simulink model "ros_deneme"  (R2021a)
settings: Solver=ode113  StartTime=0.0  StopTime=10  FixedStep=0.1  MaxStep=0.1  RelTol=1e-3
model workspace (MAT data in the model file):
  SL_ROS_VariableLengthArrays_MaxSizes.CommonInfo.ArrayTruncateAction = 'EmitWarning'
  SL_ROS_VariableLengthArrays_MaxSizes.MsgTypeMap = containers.Map
  SL_ROS_VariableLengthArrays_MaxSizes.MsgTypeMap.serialization.keys = {'sensor_msgs/Image'}
  SL_ROS_VariableLengthArrays_MaxSizes.MsgTypeMap.serialization.values{1}(1).PropertyName = 'Data'
  SL_ROS_VariableLengthArrays_MaxSizes.MsgTypeMap.serialization.values{1}(1).DataType = 'uint8'
  SL_ROS_VariableLengthArrays_MaxSizes.MsgTypeMap.serialization.values{1}(1).MaxLength = 921600
  SL_ROS_VariableLengthArrays_MaxSizes.MsgTypeMap.serialization.values{1}(2).PropertyName = 'Encoding'
  SL_ROS_VariableLengthArrays_MaxSizes.MsgTypeMap.serialization.values{1}(2).DataType = 'uint8'
  SL_ROS_VariableLengthArrays_MaxSizes.MsgTypeMap.serialization.values{1}(2).MaxLength = 128
  SL_ROS_VariableLengthArrays_MaxSizes.MsgTypeMap.serialization.uniformity = 0
  SL_ROS_VariableLengthArrays_MaxSizes.MsgTypeMap.serialization.keyType = 'char'
  SL_ROS_VariableLengthArrays_MaxSizes.MsgTypeMap.serialization.valueType = 'any'
values from neighbouring files (symbols this model uses):
  A_Lat_F = [ Yb/V        Yp/V            (Yr/V)-1       9.81/V ... (first row only)    [modelCode.m]
  A_Long_F = [ Xu            Xw            0            -9.81 ... (first row only)    [modelCode.m]
  B_Lat_F = [ 0           Y_trim_r/V ... (first row only)    [modelCode.m]
  B_Long_F = [ Z_trim_e ... (first row only)    [modelCode.m]
  V = 85    [modelCode.m]
undefined symbols (not defined in the file or in its folder): ModelName, ModelName_SL_Info, Pose
libraries: robotlib x6, pid_lib x3, robotcorelib x1
settings Model: Creator=ommda  LastModifiedBy=lambdavary
settings SolverCC: AlgebraicLoopSolver=TrustRegion
settings DebuggingCC: SFMachineParentedDataDiag=warning

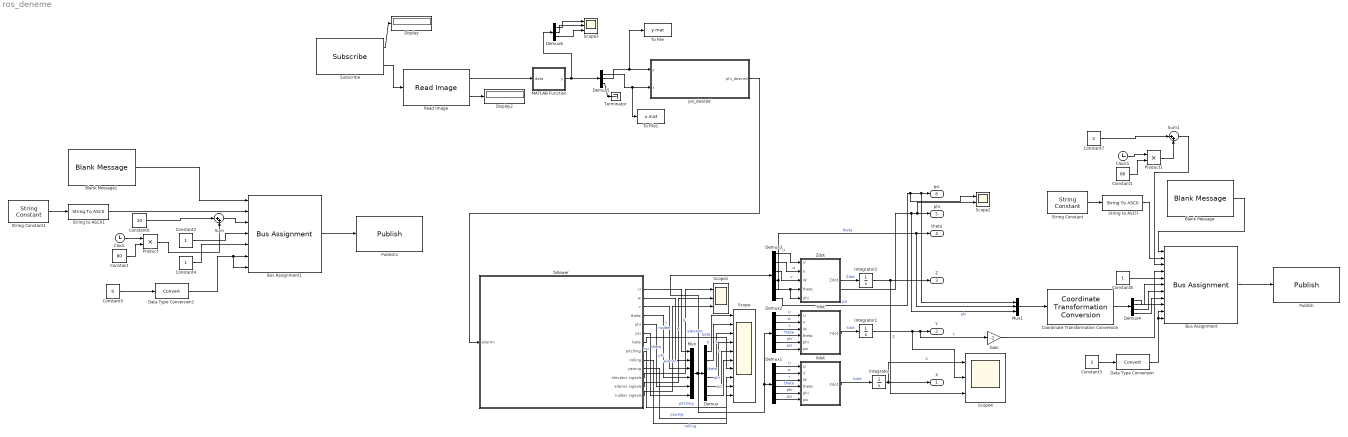
== system ros_deneme ==
  Blank Message : robotlib/Blank Message  messageClass=Message  entityType=gazebo_msgs/ModelState  messageType=gazebo_msgs/ModelState  SampleTime=inf  legacyBusStruct=off
  Blank Message1 : robotlib/Blank Message  messageClass=Message  entityType=gazebo_msgs/ModelState  messageType=gazebo_msgs/ModelState  SampleTime=inf  legacyBusStruct=off
  Bus Assignment : BusAssignment  AssignedSignals=ModelName,Pose.Position.X,Pose.Position.Y,Pose.Position.Z,Pose.Orientation.X,Pose.Orientation.Y,Pose.Orientation.Z,Pose.Orientation.W,ModelName_SL_Info.CurrentLength,ModelName_SL_Info.ReceivedLength
  Bus Assignment1 : BusAssignment  AssignedSignals=ModelName,Pose.Position.X,Pose.Position.Y,Pose.Position.Z,ModelName_SL_Info.CurrentLength,ModelName_SL_Info.ReceivedLength
  Clock : Clock
  Clock1 : Clock
  Constant : Constant  Value=80
  Constant1 : Constant  Value=80
  Constant2 : Constant
  Constant3 : Constant  Value=3
  Constant4 : Constant
  Constant5 : Constant  Value=6
  Constant6 : Constant  Value=10
  Constant7 : Constant  Value=2
  Constant8 : Constant
  Coordinate Transformation Conversion : robotcorelib/Coordinate Transformation Conversion  InputRepresentation=Euler Angles  InputEulerSequence=ZYX  ShowTrVecInputPort=on  OutputRepresentation=Quaternion  OutputEulerSequence=ZYX  ShowTrVecOutputPort=on  SimulateUsing=Interpreted execution
      settings: SourceProductBaseCode=NV,RO,RR,UV
  Data Type Conversion : DataTypeConversion
  Data Type Conversion1 : DataTypeConversion
  Demux{,1..3} (4 alike) : Demux  Outputs=6
  Demux4 : Demux
  Demux5 : Demux  Outputs=3
  Demux6 : Demux  Outputs=3
  Display : Display
  Display2 : Display
  Gain : Gain  Gain=-1
  Integrator : Integrator
  Integrator1 : Integrator
  Integrator2 : Integrator
  MATLAB Function : MATLAB Function  TreatAsAtomicUnit=on
  Mux : Mux  Inputs=6
  Mux1 : Mux  Inputs=3
  Product : Product
  Product1 : Product
  Publish : robotlib/Publish  topicSource=Select from ROS network  topic=/gazebo/set_model_state  messageType=gazebo_msgs/ModelState  legacyBusStruct=off  messageQueueLength=1
  Publish1 : robotlib/Publish  topicSource=Select from ROS network  topic=/gazebo/set_model_state  messageType=gazebo_msgs/ModelState  legacyBusStruct=off  messageQueueLength=1
  Read Image : robotlib/Read Image  MaximumImageSize=[480, 640]  ImageEncoding=rgb8  ShowAlphaOutput=off  ShowErrorCodeOutput=on  VariableSizeOutputs=off
      settings: SourceProductBaseCode=RR
  Scope : Scope  NumInputPorts=10
  Scope1 : Scope  NumInputPorts=3
  Scope2 : Scope  NumInputPorts=2
  Scope3 : Scope  NumInputPorts=3
  Scope4 : Scope  NumInputPorts=3
  String Constant : StringConstant  String="\"yau\""
  String Constant1 : StringConstant  String="\"tanker\""
  String to ASCII : StringToASCII  OutputVectorSize=128
  String to ASCII1 : StringToASCII  OutputVectorSize=128
  Subscribe : robotlib/Subscribe  topicSource=Select from ROS network  topic=/camera/image_raw  messageType=sensor_msgs/Image  SampleTime=-1  legacyBusStruct=off  messageQueueLength=1
  Sum : Sum  Inputs=|++
  Sum1 : Sum  Inputs=|++
  Terminator : Terminator
  To File : ToFile  Filename=y.mat
  To File1 : ToFile  Filename=x.mat
  Xdot : Subsystem
  Ydot : Subsystem
  Zdot : Subsystem
  follower : Subsystem
      mask Display: image('D:\Downloads\1200px-Yaw_Axis_Corrected.svg.png'); % Use "Edit Image" on toolstrip to change.
  psi_desired : Subsystem
  X : Outport
  Y : Outport  Port=2
  Z : Outport  Port=3
  theta : Outport  Port=4
  phi : Outport  Port=5
  psi : Outport  Port=6
  wires:
  Demux2/3 -> Ydot/3(W)  "v"
  Demux2/2 -> Ydot/2(V)  "w"
  follower/3(v) -> Mux/3  "v"
  Zdot/1(Zdot) -> Integrator2/1  "Zdot"
  Ydot/1(Ydot) -> Integrator1/1  "Ydot"
  Demux2/4 -> Ydot/4(theta)  "theta"
  Demux/3 -> Scope/3  "v"
  follower/7(beta) -> Scope/7  "beta"
  follower/1(U) -> Mux/1  "U"
  Demux3/5 -> Mux1/3, Scope2/2, phi/1, Zdot/5(phi)  "phi"
  Demux3/1 -> Zdot/1(U)  "U"
  Integrator/1 -> Scope4/1, X/1  "X"
  Demux1/3 -> Xdot/3(W)  "v"
  Mux/1 -> Demux2/1, Demux1/1, Demux3/1, Demux/1
  Demux1/6 -> Xdot/6(psi)  "psi"
  follower/5(phi) -> Mux/5  "phi"
  Integrator1/1 -> Scope4/2, Gain/1, Y/1  "Y"
  Integrator2/1 -> Scope4/3, Z/1  "Z"
  Demux1/2 -> Xdot/2(V)  "w"
  Demux2/5 -> Ydot/5(phi)  "phi"
  Demux1/4 -> Xdot/4(theta)  "theta"
  Demux2/6 -> Ydot/6(psi)  "psi"
  Demux/1 -> Scope/1  "U"
  Demux2/1 -> Ydot/1(U)  "U"
  follower/4(theta) -> Mux/4  "theta"
  Demux1/5 -> Xdot/5(phi)  "phi"
  Demux3/4 -> Mux1/2, theta/1, Zdot/4(theta)  "theta"
  Demux3/2 -> Zdot/2(V)  "w"
  Demux1/1 -> Xdot/1(U)  "U"
  follower/12(aileron signals) -> Scope1/2  "aileron"
  follower/8(pitching) -> Scope/8  "pitching"
  follower/9(rolling) -> Scope/9  "rolling"
  follower/11("elevator signals ") -> Scope1/1  "elevator"
  Demux/5 -> Scope/5  "phi"
  follower/13(rudder signals) -> Scope1/3  "rudder"
  Demux/6 -> Scope/6  "psi"
  Xdot/1(Xdot) -> Integrator/1  "Xdot"
  follower/6(psi) -> Mux/6  "psi"
  Demux/2 -> Scope/2  "w"
  follower/2(w) -> Mux/2  "w"
  follower/10(yawing) -> Scope/10  "yawing"
  Demux/4 -> Scope/4  "theta"
  Demux3/3 -> Zdot/3(W)  "v"
  Demux3/6 -> Scope2/1, Mux1/1, psi/1  "psi"
  Bus Assignment/1 -> Publish/1
  String Constant/1 -> String to ASCII/1
  String to ASCII/1 -> Bus Assignment/2
  Constant3/1 -> Data Type Conversion/1
  Blank Message/1 -> Bus Assignment/1
  Coordinate Transformation Conversion/1 -> Demux4/1
  Demux4/1 -> Bus Assignment/9
  Demux4/2 -> Bus Assignment/6
  Demux4/3 -> Bus Assignment/7
  Demux4/4 -> Bus Assignment/8
  Data Type Conversion/1 -> Bus Assignment/11, Bus Assignment/10
  Mux1/1 -> Coordinate Transformation Conversion/1
  Clock1/1 -> Product1/1
  Constant1/1 -> Product1/2
  Constant7/1 -> Sum1/1
  Product1/1 -> Sum1/2
  Sum1/1 -> Bus Assignment/3
  Constant8/1 -> Bus Assignment/5
  Constant4/1 -> Bus Assignment1/5
  Sum/1 -> Bus Assignment1/3
  Constant2/1 -> Bus Assignment1/4
  Constant/1 -> Product/2
  Constant5/1 -> Data Type Conversion1/1
  Data Type Conversion1/1 -> Bus Assignment1/7, Bus Assignment1/6
  String Constant1/1 -> String to ASCII1/1
  Clock/1 -> Product/1
  Constant6/1 -> Sum/1
  Blank Message1/1 -> Bus Assignment1/1
  Bus Assignment1/1 -> Publish1/1
  String to ASCII1/1 -> Bus Assignment1/2
  Product/1 -> Sum/2
  Read Image/1 -> MATLAB Function/1(data)
  Read Image/2 -> Display2/1
  MATLAB Function/1(y) -> Demux6/1, Demux5/1
  Subscribe/2 -> Read Image/1
  Subscribe/1 -> Display/1
  Demux5/2 -> To File/1, psi_desired/1(y)
  Demux5/3 -> Terminator/1
  Demux5/1 -> To File1/1, psi_desired/2(x)
  psi_desired/1(phi_desired) -> follower/1(aileron)
  Gain/1 -> Bus Assignment/4
  Demux6/1 -> Scope3/1
  Demux6/2 -> Scope3/2
  Demux6/3 -> Scope3/3

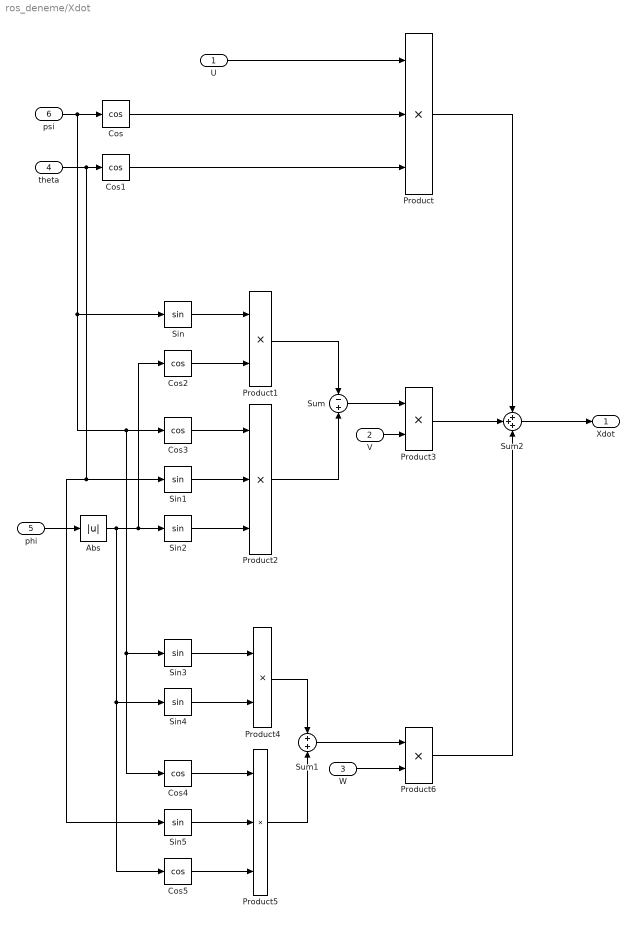
== system ros_deneme/Xdot ==
  U : Inport
  V : Inport  Port=2
  W : Inport  Port=3
  theta : Inport  Port=4
  phi : Inport  Port=5
  psi : Inport  Port=6
  Abs : Abs
  Cos{,1..5} (6 alike) : Trigonometry  Operator=cos
  Product : Product  Inputs=3
  Product{1,3..4,6} (4 alike) : Product
  Product2 : Product  Inputs=3
  Product5 : Product  Inputs=3
  Sin{,1..5} (6 alike) : Trigonometry
  Sum : Sum  Inputs=-+
  Sum1 : Sum
  Sum2 : Sum  Inputs=+++
  Xdot : Outport
  wires:
  psi/1 -> Cos/1, Sin/1, Sin3/1, Cos4/1, Cos3/1
  phi/1 -> Abs/1
  theta/1 -> Sin1/1, Sin5/1, Cos1/1
  U/1 -> Product/1
  Cos/1 -> Product/2
  Cos1/1 -> Product/3
  Abs/1 -> Cos2/1, Sin2/1, Sin4/1, Cos5/1
  Sin/1 -> Product1/1
  Cos2/1 -> Product1/2
  Cos3/1 -> Product2/1
  Sin1/1 -> Product2/2
  Sin2/1 -> Product2/3
  Product1/1 -> Sum/1
  Product2/1 -> Sum/2
  Sum/1 -> Product3/1
  V/1 -> Product3/2
  Sin3/1 -> Product4/1
  Sin4/1 -> Product4/2
  Cos4/1 -> Product5/1
  Sin5/1 -> Product5/2
  Cos5/1 -> Product5/3
  Product4/1 -> Sum1/1
  Product5/1 -> Sum1/2
  Sum1/1 -> Product6/1
  W/1 -> Product6/2
  Product3/1 -> Sum2/2
  Product/1 -> Sum2/1
  Product6/1 -> Sum2/3
  Sum2/1 -> Xdot/1

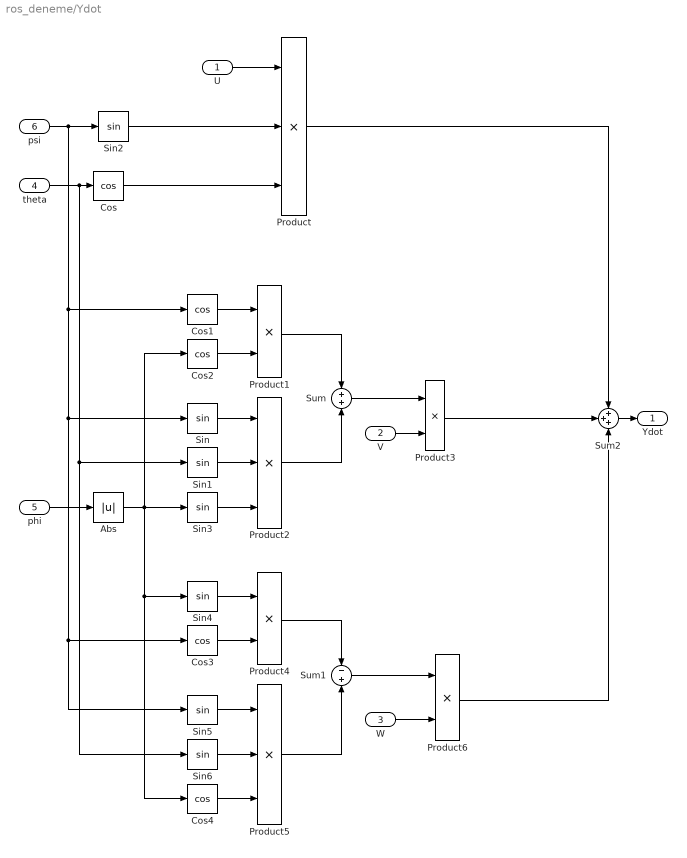
== system ros_deneme/Ydot ==
  U : Inport
  V : Inport  Port=2
  W : Inport  Port=3
  theta : Inport  Port=4
  phi : Inport  Port=5
  psi : Inport  Port=6
  Abs : Abs
  Cos{,1..4} (5 alike) : Trigonometry  Operator=cos
  Product : Product  Inputs=3
  Product{1,3..4,6} (4 alike) : Product
  Product2 : Product  Inputs=3
  Product5 : Product  Inputs=3
  Sin{,1..6} (7 alike) : Trigonometry
  Sum : Sum
  Sum1 : Sum  Inputs=-+
  Sum2 : Sum  Inputs=+++
  Ydot : Outport
  wires:
  psi/1 -> Cos1/1, Sin5/1, Cos3/1, Sin/1, Sin2/1
  theta/1 -> Sin1/1, Sin6/1, Cos/1
  Cos/1 -> Product/3
  Sin2/1 -> Product/2
  U/1 -> Product/1
  phi/1 -> Abs/1
  Abs/1 -> Sin3/1, Cos4/1, Sin4/1, Cos2/1
  Cos1/1 -> Product1/1
  Cos2/1 -> Product1/2
  Sin/1 -> Product2/1
  Sin1/1 -> Product2/2
  Sin3/1 -> Product2/3
  Product1/1 -> Sum/1
  Product2/1 -> Sum/2
  Sum/1 -> Product3/1
  V/1 -> Product3/2
  Sin4/1 -> Product4/1
  Cos3/1 -> Product4/2
  Sin5/1 -> Product5/1
  Sin6/1 -> Product5/2
  Cos4/1 -> Product5/3
  Product4/1 -> Sum1/1
  Product5/1 -> Sum1/2
  Sum1/1 -> Product6/1
  W/1 -> Product6/2
  Sum2/1 -> Ydot/1
  Product3/1 -> Sum2/2
  Product/1 -> Sum2/1
  Product6/1 -> Sum2/3

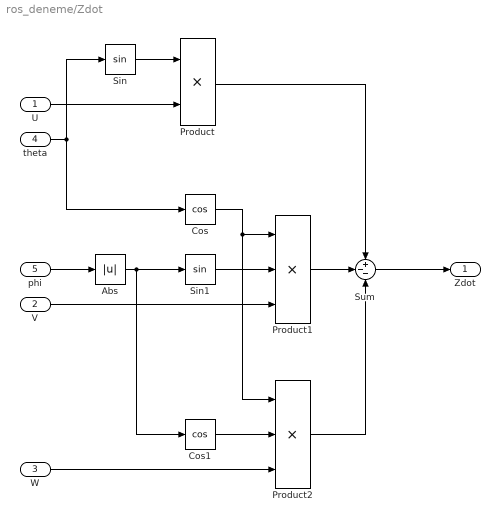
== system ros_deneme/Zdot ==
  U : Inport
  V : Inport  Port=2
  W : Inport  Port=3
  theta : Inport  Port=4
  phi : Inport  Port=5
  Abs : Abs
  Cos : Trigonometry  Operator=cos
  Cos1 : Trigonometry  Operator=cos
  Product : Product
  Product1 : Product  Inputs=3
  Product2 : Product  Inputs=3
  Sin : Trigonometry
  Sin1 : Trigonometry
  Sum : Sum  Inputs=+--
  Zdot : Outport
  wires:
  theta/1 -> Cos/1, Sin/1
  Sin/1 -> Product/1
  U/1 -> Product/2
  phi/1 -> Abs/1
  Abs/1 -> Cos1/1, Sin1/1
  Cos/1 -> Product2/1, Product1/1
  Sin1/1 -> Product1/2
  V/1 -> Product1/3
  Cos1/1 -> Product2/2
  W/1 -> Product2/3
  Product1/1 -> Sum/2
  Product/1 -> Sum/1
  Product2/1 -> Sum/3
  Sum/1 -> Zdot/1

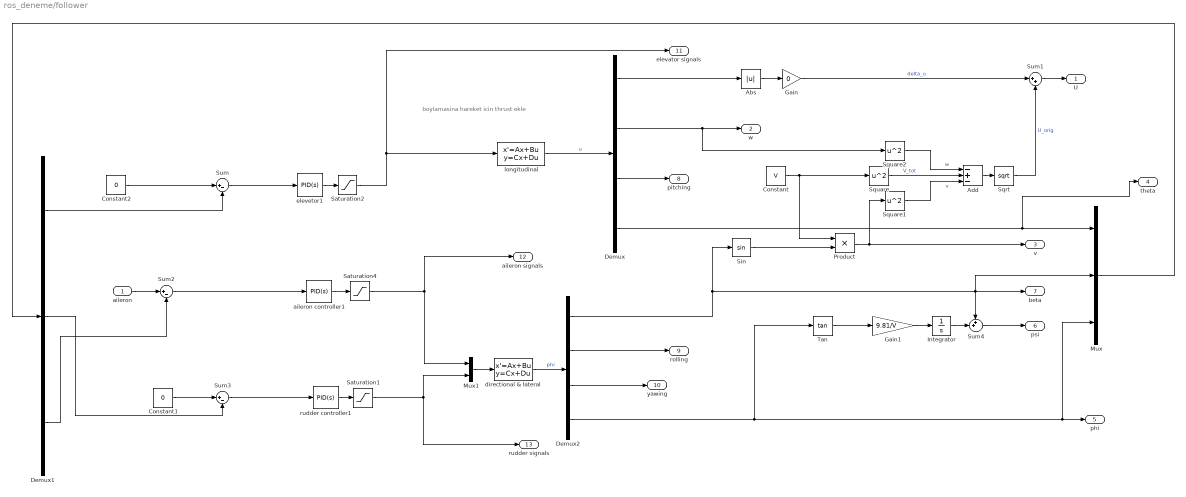
== system ros_deneme/follower ==
  note: boylamasina hareket icin thrust ekle
  aileron : Inport
  Abs : Abs
  Add : Sum  Inputs=-+-
  Constant : Constant  Value=V
  Constant1 : Constant  Value=0
  Constant2 : Constant  Value=0
  Demux : Demux
  Demux1 : Demux  Outputs=3
  Demux2 : Demux
  Gain : Gain  Gain=0
  Gain1 : Gain  Gain=9.81/V
  Integrator : Integrator
  Mux : Mux  Inputs=3
  Mux1 : Mux  Inputs=2
  Product : Product
  Saturation1 : Saturate  UpperLimit=0.523599  LowerLimit=-0.523599
  Saturation2 : Saturate  UpperLimit=0.523599  LowerLimit=-0.523599
  Saturation4 : Saturate  UpperLimit=0.523599  LowerLimit=-0.523599
  Sin : Trigonometry
  Sqrt : Sqrt  SaturateOnIntegerOverflow=on
  Square : Math  Operator=square  SaturateOnIntegerOverflow=on
  Square1 : Math  Operator=square  SaturateOnIntegerOverflow=on
  Square2 : Math  Operator=square  SaturateOnIntegerOverflow=on
  Sum : Sum  Inputs=|+-
  Sum1 : Sum  Inputs=|++
  Sum2 : Sum  Inputs=|+-
  Sum3 : Sum  Inputs=|+-
  Sum4 : Sum  Inputs=++|
  Tan : Trigonometry  Operator=tan
  aileron controller1 : pid_lib/PID Controller  Controller=PID  Form=Parallel  TimeDomain=Continuous-time  UseExternalTs=off  SampleTime=-1  IntegratorMethod=Forward Euler  FilterMethod=Forward Euler  ControllerParametersSource=internal  P=1.23740502206763  I=2.08998402399655  D=0.0648471425518328  UseFilter=on  N=17.8373087295252  TunerSelectOption=Transfer Function Based (PID Tuner App)  InitialConditionSource=internal  InitialConditionForIntegrator=0  InitialConditionForFilter=0  DifferentiatorICPrevScaledInput=0  ExternalReset=none  TrackingMode=off  Kt=1  LimitOutput=off  SatLimitsSource=internal  UpperSaturationLimit=inf  LowerSaturationLimit=-inf  LinearizeAsGain=on  AntiWindupMode=none  Kb=1  POutMin=[]  POutMax=[]  IOutMin=[]  IOutMax=[]  DOutMin=[]  DOutMax=[]  NOutMin=[]  NOutMax=[]  SumOutMin=[]  SumOutMax=[]  SaturationOutMin=[]  SaturationOutMax=[]  PParamMin=[]  PParamMax=[]  IParamMin=[]  IParamMax=[]  DParamMin=[]  DParamMax=[]  NParamMin=[]  NParamMax=[]  KbParamMin=[]  KbParamMax=[]  KtParamMin=[]  KtParamMax=[]  KbOutMin=[]  KbOutMax=[]  KtOutMin=[]  KtOutMax=[]  IntegratorOutMin=[]  IntegratorOutMax=[]  FilterOutMin=[]  FilterOutMax=[]  SumI1OutMin=[]  SumI1OutMax=[]  SumI2OutMin=[]  SumI2OutMax=[]  SumI3OutMin=[]  SumI3OutMax=[]  SumI4OutMin=[]  SumI4OutMax=[]  SumDOutMin=[]  SumDOutMax=[]  DifferentiatorOutMin=[]  DifferentiatorOutMax=[]  FilterDiffOutCoefMin=[]  FilterDiffOutCoefMax=[]  ReciprocalOutMin=[]  ReciprocalOutMax=[]  SumDenOutMin=[]  SumDenOutMax=[]  SumNumOutMin=[]  SumNumOutMax=[]  DivideOutMin=[]  DivideOutMax=[]  UdiffTsProdOutMin=[]  UdiffTsProdOutMax=[]  NTsProdOutMin=[]  NTsProdOutMax=[]  UintegralTsProdOutMin=[]  UintegralTsProdOutMax=[]  UngainTsProdOutMin=[]  UngainTsProdOutMax=[]  IntegratorContinuousStateAttributes=''  IntegratorStateMustResolveToSignalObject=off  IntegratorRTWStateStorageClass=Auto  FilterContinuousStateAttributes=''  FilterStateMustResolveToSignalObject=off  FilterRTWStateStorageClass=Auto  ParallelPVariant=InternalParameters  IdealPVariant=Disabled  IVariant=InternalParameters  DVariant=InternalParameters  IntegratorVariant=Continuous  SatVariant=Disabled  AWVariant=Passthrough  PCopyVariant=Disabled  TRVariant=Disabled  FdbkBlocksVariant=Forward  IdealPFdbkVariant=Disabled  SatFdbkVariant=Disabled  DerivativeFilterVariant=ContFilter  NVariant=InternalParameters  NCopyVariant=Disabled  FilterICVariant=InternalICsFilter  IntegratorICVariant=InternalICs  ExternalResetVariant=Disabled  TRSumVariant=Passthrough  SumFdbkVariant=Disabled  SumVariant=Sum_PID  TsampFilterVariant=InternalTs  TsampNgainVariant=Passthrough  TsampIntegralVariant=Passthrough  ExternalSaturationOutDataTypeStr=Inherit: Same as second input
  directional & lateral : StateSpace  A=A_Lat_F  B=B_Lat_F  C=eye(4)  D=[0 0; 0 0; 0 0; 0 0]  InitialCondition=0
  elevetor1 : pid_lib/PID Controller  Controller=PID  Form=Parallel  TimeDomain=Continuous-time  UseExternalTs=off  SampleTime=-1  IntegratorMethod=Forward Euler  FilterMethod=Forward Euler  ControllerParametersSource=internal  P=-0.804617234816433  I=-0.625801703536542  D=-0.0580928336585526  UseFilter=on  N=515.621985271107  TunerSelectOption=Transfer Function Based (PID Tuner App)  InitialConditionSource=internal  InitialConditionForIntegrator=0  InitialConditionForFilter=0  DifferentiatorICPrevScaledInput=0  ExternalReset=none  TrackingMode=off  Kt=1  LimitOutput=off  SatLimitsSource=internal  UpperSaturationLimit=inf  LowerSaturationLimit=-inf  LinearizeAsGain=on  AntiWindupMode=none  Kb=1  POutMin=[]  POutMax=[]  IOutMin=[]  IOutMax=[]  DOutMin=[]  DOutMax=[]  NOutMin=[]  NOutMax=[]  SumOutMin=[]  SumOutMax=[]  SaturationOutMin=[]  SaturationOutMax=[]  PParamMin=[]  PParamMax=[]  IParamMin=[]  IParamMax=[]  DParamMin=[]  DParamMax=[]  NParamMin=[]  NParamMax=[]  KbParamMin=[]  KbParamMax=[]  KtParamMin=[]  KtParamMax=[]  KbOutMin=[]  KbOutMax=[]  KtOutMin=[]  KtOutMax=[]  IntegratorOutMin=[]  IntegratorOutMax=[]  FilterOutMin=[]  FilterOutMax=[]  SumI1OutMin=[]  SumI1OutMax=[]  SumI2OutMin=[]  SumI2OutMax=[]  SumI3OutMin=[]  SumI3OutMax=[]  SumI4OutMin=[]  SumI4OutMax=[]  SumDOutMin=[]  SumDOutMax=[]  DifferentiatorOutMin=[]  DifferentiatorOutMax=[]  FilterDiffOutCoefMin=[]  FilterDiffOutCoefMax=[]  ReciprocalOutMin=[]  ReciprocalOutMax=[]  SumDenOutMin=[]  SumDenOutMax=[]  SumNumOutMin=[]  SumNumOutMax=[]  DivideOutMin=[]  DivideOutMax=[]  UdiffTsProdOutMin=[]  UdiffTsProdOutMax=[]  NTsProdOutMin=[]  NTsProdOutMax=[]  UintegralTsProdOutMin=[]  UintegralTsProdOutMax=[]  UngainTsProdOutMin=[]  UngainTsProdOutMax=[]  IntegratorContinuousStateAttributes=''  IntegratorStateMustResolveToSignalObject=off  IntegratorRTWStateStorageClass=Auto  FilterContinuousStateAttributes=''  FilterStateMustResolveToSignalObject=off  FilterRTWStateStorageClass=Auto  ParallelPVariant=InternalParameters  IdealPVariant=Disabled  IVariant=InternalParameters  DVariant=InternalParameters  IntegratorVariant=Continuous  SatVariant=Disabled  AWVariant=Passthrough  PCopyVariant=Disabled  TRVariant=Disabled  FdbkBlocksVariant=Forward  IdealPFdbkVariant=Disabled  SatFdbkVariant=Disabled  DerivativeFilterVariant=ContFilter  NVariant=InternalParameters  NCopyVariant=Disabled  FilterICVariant=InternalICsFilter  IntegratorICVariant=InternalICs  ExternalResetVariant=Disabled  TRSumVariant=Passthrough  SumFdbkVariant=Disabled  SumVariant=Sum_PID  TsampFilterVariant=InternalTs  TsampNgainVariant=Passthrough  TsampIntegralVariant=Passthrough  ExternalSaturationOutDataTypeStr=Inherit: Same as second input
  longitudinal : StateSpace  A=A_Long_F  B=B_Long_F  C=eye(4)  D=[0;0;0;0]  InitialCondition=0
  rudder controller1 : pid_lib/PID Controller  Controller=PID  Form=Parallel  TimeDomain=Continuous-time  UseExternalTs=off  SampleTime=-1  IntegratorMethod=Forward Euler  FilterMethod=Forward Euler  ControllerParametersSource=internal  P=1.48843500027863  I=5.15386062628497  D=0.106478981231435  UseFilter=on  N=983.424476419589  TunerSelectOption=Transfer Function Based (PID Tuner App)  InitialConditionSource=internal  InitialConditionForIntegrator=0  InitialConditionForFilter=0  DifferentiatorICPrevScaledInput=0  ExternalReset=none  TrackingMode=off  Kt=1  LimitOutput=off  SatLimitsSource=internal  UpperSaturationLimit=inf  LowerSaturationLimit=-inf  LinearizeAsGain=on  AntiWindupMode=none  Kb=1  POutMin=[]  POutMax=[]  IOutMin=[]  IOutMax=[]  DOutMin=[]  DOutMax=[]  NOutMin=[]  NOutMax=[]  SumOutMin=[]  SumOutMax=[]  SaturationOutMin=[]  SaturationOutMax=[]  PParamMin=[]  PParamMax=[]  IParamMin=[]  IParamMax=[]  DParamMin=[]  DParamMax=[]  NParamMin=[]  NParamMax=[]  KbParamMin=[]  KbParamMax=[]  KtParamMin=[]  KtParamMax=[]  KbOutMin=[]  KbOutMax=[]  KtOutMin=[]  KtOutMax=[]  IntegratorOutMin=[]  IntegratorOutMax=[]  FilterOutMin=[]  FilterOutMax=[]  SumI1OutMin=[]  SumI1OutMax=[]  SumI2OutMin=[]  SumI2OutMax=[]  SumI3OutMin=[]  SumI3OutMax=[]  SumI4OutMin=[]  SumI4OutMax=[]  SumDOutMin=[]  SumDOutMax=[]  DifferentiatorOutMin=[]  DifferentiatorOutMax=[]  FilterDiffOutCoefMin=[]  FilterDiffOutCoefMax=[]  ReciprocalOutMin=[]  ReciprocalOutMax=[]  SumDenOutMin=[]  SumDenOutMax=[]  SumNumOutMin=[]  SumNumOutMax=[]  DivideOutMin=[]  DivideOutMax=[]  UdiffTsProdOutMin=[]  UdiffTsProdOutMax=[]  NTsProdOutMin=[]  NTsProdOutMax=[]  UintegralTsProdOutMin=[]  UintegralTsProdOutMax=[]  UngainTsProdOutMin=[]  UngainTsProdOutMax=[]  IntegratorContinuousStateAttributes=''  IntegratorStateMustResolveToSignalObject=off  IntegratorRTWStateStorageClass=Auto  FilterContinuousStateAttributes=''  FilterStateMustResolveToSignalObject=off  FilterRTWStateStorageClass=Auto  ParallelPVariant=InternalParameters  IdealPVariant=Disabled  IVariant=InternalParameters  DVariant=InternalParameters  IntegratorVariant=Continuous  SatVariant=Disabled  AWVariant=Passthrough  PCopyVariant=Disabled  TRVariant=Disabled  FdbkBlocksVariant=Forward  IdealPFdbkVariant=Disabled  SatFdbkVariant=Disabled  DerivativeFilterVariant=ContFilter  NVariant=InternalParameters  NCopyVariant=Disabled  FilterICVariant=InternalICsFilter  IntegratorICVariant=InternalICs  ExternalResetVariant=Disabled  TRSumVariant=Passthrough  SumFdbkVariant=Disabled  SumVariant=Sum_PID  TsampFilterVariant=InternalTs  TsampNgainVariant=Passthrough  TsampIntegralVariant=Passthrough  ExternalSaturationOutDataTypeStr=Inherit: Same as second input
  U : Outport
  w : Outport  Port=2
  v : Outport  Port=3
  theta : Outport  Port=4
  phi : Outport  Port=5
  psi : Outport  Port=6
  beta : Outport  Port=7
  pitching : Outport  Port=8
  rolling : Outport  Port=9
  yawing : Outport  Port=10
  "elevator signals " : Outport  Port=11
  aileron signals : Outport  Port=12
  rudder signals : Outport  Port=13
  wires:
  Sin/1 -> Product/2
  Constant/1 -> Product/1, Square/1
  Product/1 -> Square1/1, v/1
  Abs/1 -> Gain/1
  Gain/1 -> Sum1/1  "delta_u"
  Square/1 -> Add/2  "V_tot"
  Square2/1 -> Add/1  "w"
  Square1/1 -> Add/3  "v"
  Add/1 -> Sqrt/1
  Sqrt/1 -> Sum1/2  "U_orig"
  Sum1/1 -> U/1
  Demux/2 -> Square2/1, w/1
  Saturation2/1 -> longitudinal/1, "elevator signals "/1
  Demux/1 -> Abs/1
  Demux/3 -> pitching/1
  Demux2/1 -> beta/1, Mux/2, Sum4/1, Sin/1
  Demux2/3 -> yawing/1
  Tan/1 -> Gain1/1
  Gain1/1 -> Integrator/1
  Integrator/1 -> Sum4/2
  Demux2/4 -> Tan/1, Mux/3, phi/1
  Mux/1 -> Demux1/1
  longitudinal/1 -> Demux/1  "u"
  Saturation1/1 -> rudder signals/1, Mux1/2
  Saturation4/1 -> Mux1/1, aileron signals/1
  Mux1/1 -> directional & lateral/1
  directional & lateral/1 -> Demux2/1  "phi"
  Demux1/3 -> Sum2/2
  aileron/1 -> Sum2/1
  Demux1/2 -> Sum3/2
  Constant1/1 -> Sum3/1
  Demux1/1 -> Sum/2
  Constant2/1 -> Sum/1
  Sum/1 -> elevetor1/1
  Sum3/1 -> rudder controller1/1
  Sum2/1 -> aileron controller1/1
  Sum4/1 -> psi/1
  elevetor1/1 -> Saturation2/1
  aileron controller1/1 -> Saturation4/1
  rudder controller1/1 -> Saturation1/1
  Demux2/2 -> rolling/1
  Demux/4 -> theta/1, Mux/1

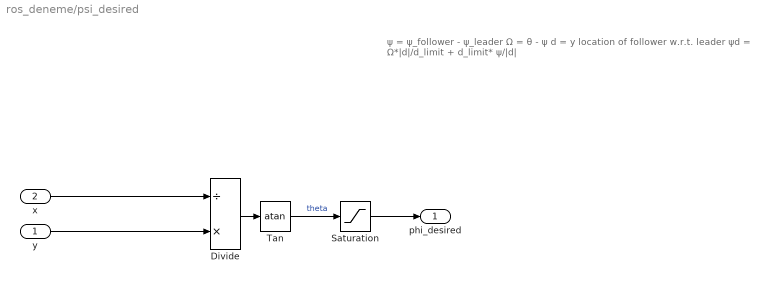
== system ros_deneme/psi_desired ==
  note: ψ = ψ_follower - ψ_leader
      | Ω = θ - ψ
      | d = y location of follower w.r.t. leader
      |
      | ψd = Ω*|d|/d_limit + d_limit* ψ/|d|
  y : Inport
  x : Inport  Port=2
  Divide : Product  Inputs=/*
  Saturation : Saturate  UpperLimit=1.0472  LowerLimit=-1.0472
  Tan : Trigonometry  Operator=atan
  phi_desired : Outport
  wires:
  y/1 -> Divide/2
  x/1 -> Divide/1
  Divide/1 -> Tan/1
  Saturation/1 -> phi_desired/1
  Tan/1 -> Saturation/1  "theta"

== matlab function ros_deneme/MATLAB Function ==
  data: y output; data input
function y = fcn(data)

[centersDark,radiiDark] = imfindcircles(data,[10 300],'ObjectPolarity','dark', 'Sensitivity',0.92);

if ~isempty(centersDark)
    xPos = -5.983*10^-7*radiiDark(1)^5 + 0.0001086*radiiDark(1)^4 - 0.00788*radiiDark(1)^3 + 0.292*radiiDark(1)^2 - 5.812*radiiDark(1) + 59;
    yPos = (320-centersDark(1))/(2*radiiDark(1));
    zPos = (240-centersDark(2))/(1.5*radiiDark(1));
else
    xPos = 0.001;
    yPos = 0.001;
    zPos = 0.001;
end
if ~isempty(centersDark) && centersDark(1) < 320
    yPos = -yPos;
end
if ~isempty(centersDark) && centersDark(2) > 240
    zPos = -zPos;
end
y = [ xPos yPos zPos ];
